simulink library "SEMACE1_IN"  (R2021b)
settings: Solver=VariableStepAuto  StartTime=0.0  StopTime=10.0  RelTol=1e-3
values from neighbouring files (symbols this model uses):
  dataSEMACE = 60.0    [applicationDD.sldd]    (also in dataSEMACE.mat = ; dataSEMACE_DD.sldd)
settings Model: Creator=ACH  LastModifiedBy=ACH

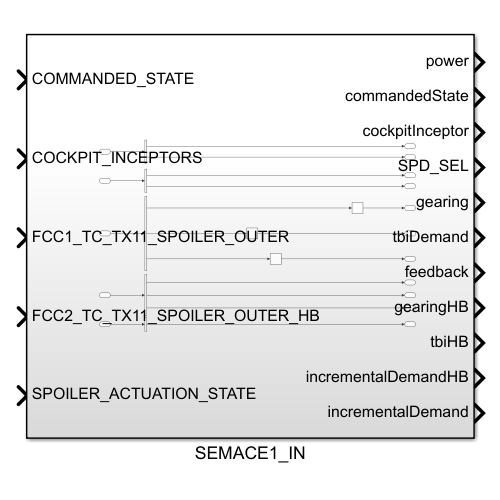
[thumbnail: Simulink's stored preview of the top-level diagram]
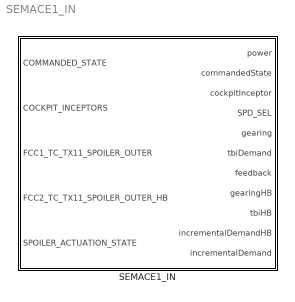
== system SEMACE1_IN ==
  SEMACE1_IN : Subsystem

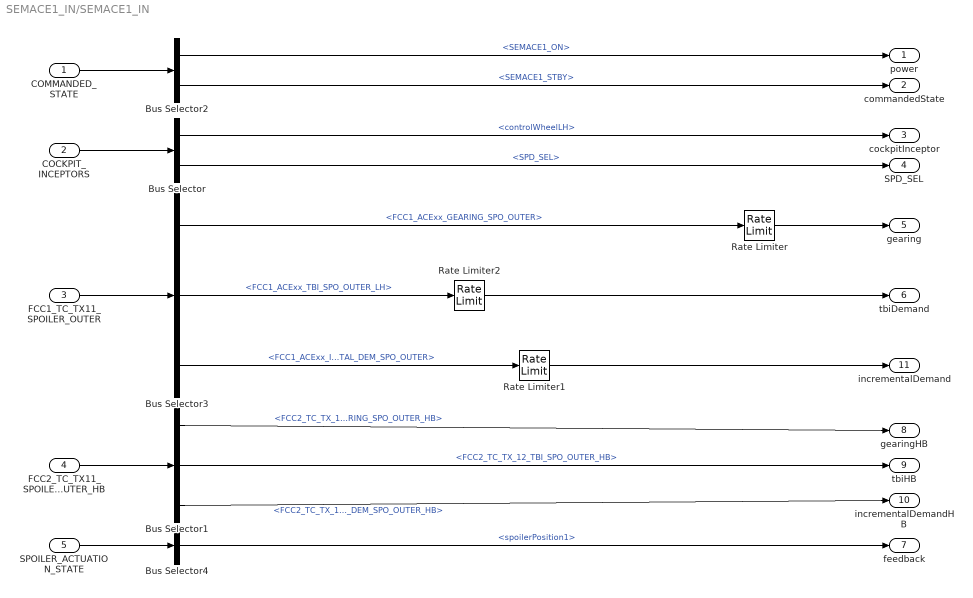
== system SEMACE1_IN/SEMACE1_IN ==
  COMMANDED_STATE : Inport  OutDataTypeStr=Bus: COMMANDED_STATE
  COCKPIT_INCEPTORS : Inport  Port=2  OutDataTypeStr=Bus: COCKPIT_INCEPTORS
  FCC1_TC_TX11_SPOILER_OUTER : Inport  Port=3  OutDataTypeStr=Bus: FCC1_TC_TX_11_SPOILER_OUTER
  FCC2_TC_TX11_SPOILER_OUTER_HB : Inport  Port=4  OutDataTypeStr=Bus: FCC2_TC_TX_11_SPOILER_OUTER_HB
  SPOILER_ACTUATION_STATE : Inport  Port=5  OutDataTypeStr=Bus: SPOILER_ACTUATION_STATE
  Bus Selector : BusSelector  OutputSignals=controlWheelLH,SPD_SEL
  Bus Selector1 : BusSelector  OutputSignals=FCC2_TC_TX_12_GEARING_SPO_OUTER_HB,FCC2_TC_TX_12_TBI_SPO_OUTER_HB,FCC2_TC_TX_12_INCREMENTAL_DEM_SPO_OUTER_HB
  Bus Selector2 : BusSelector  OutputSignals=SEMACE1_ON,SEMACE1_STBY
  Bus Selector3 : BusSelector  OutputSignals=FCC1_ACExx_GEARING_SPO_OUTER,FCC1_ACExx_TBI_SPO_OUTER_LH,FCC1_ACExx_INCREMENTAL_DEM_SPO_OUTER
  Bus Selector4 : BusSelector  OutputSignals=spoilerPosition1
  Rate Limiter : RateLimiter  RisingSlewLimit=dataSEMACE.rateLimiterGearing  FallingSlewLimit=-dataSEMACE.rateLimiterGearing  SampleTimeMode=inherited
      settings: AttributesFormatString=|
      | %<RisingSlewLimit>
      | %<FallingSlewLimit>
  Rate Limiter1 : RateLimiter  RisingSlewLimit=dataSEMACE.rateLimiterSymmetric  FallingSlewLimit=-dataSEMACE.rateLimiterSymmetric  SampleTimeMode=inherited
      settings: AttributesFormatString=|
      | %<RisingSlewLimit>
      | %<FallingSlewLimit>
  Rate Limiter2 : RateLimiter  RisingSlewLimit=dataSEMACE.rateLimiterTBI  FallingSlewLimit=-dataSEMACE.rateLimiterTBI  SampleTimeMode=inherited
      settings: AttributesFormatString=|
      | %<RisingSlewLimit>
      | %<FallingSlewLimit>
  power : Outport
  commandedState : Outport  Port=2
  cockpitInceptor : Outport  Port=3
  SPD_SEL : Outport  Port=4
  gearing : Outport  Port=5
  tbiDemand : Outport  Port=6
  feedback : Outport  Port=7
  gearingHB : Outport  Port=8
  tbiHB : Outport  Port=9
  incrementalDemandHB : Outport  Port=10
  incrementalDemand : Outport  Port=11
  wires:
  Bus Selector3/2 -> Rate Limiter2/1  "<FCC1_ACExx_TBI_SPO_OUTER_LH>"
  Bus Selector3/3 -> Rate Limiter1/1  "<FCC1_ACExx_INCREMENTAL_DEM_SPO_OUTER>"
  SPOILER_ACTUATION_STATE/1 -> Bus Selector4/1
  Bus Selector2/1 -> power/1  "<SEMACE1_ON>"
  Bus Selector4/1 -> feedback/1  "<spoilerPosition1>"
  COMMANDED_STATE/1 -> Bus Selector2/1
  FCC1_TC_TX11_SPOILER_OUTER/1 -> Bus Selector3/1
  COCKPIT_INCEPTORS/1 -> Bus Selector/1
  Bus Selector/1 -> cockpitInceptor/1  "<controlWheelLH>"
  Bus Selector3/1 -> Rate Limiter/1  "<FCC1_ACExx_GEARING_SPO_OUTER>"
  Rate Limiter/1 -> gearing/1
  Bus Selector2/2 -> commandedState/1  "<SEMACE1_STBY>"
  Bus Selector/2 -> SPD_SEL/1  "<SPD_SEL>"
  FCC2_TC_TX11_SPOILER_OUTER_HB/1 -> Bus Selector1/1
  Bus Selector1/1 -> gearingHB/1  "<FCC2_TC_TX_12_GEARING_SPO_OUTER_HB>"
  Bus Selector1/2 -> tbiHB/1  "<FCC2_TC_TX_12_TBI_SPO_OUTER_HB>"
  Bus Selector1/3 -> incrementalDemandHB/1  "<FCC2_TC_TX_12_INCREMENTAL_DEM_SPO_OUTER_HB>"
  Rate Limiter2/1 -> tbiDemand/1
  Rate Limiter1/1 -> incrementalDemand/1
